simulink library "inp"  (R2021b)
settings: Solver=VariableStepAuto  StartTime=0.0  StopTime=10.0  RelTol=1e-3
undefined symbols (not defined in the file): C_TASK_5MS_S, FALSE, KINP_AcoreReadyToSlp_flg_ovrdflg, KINP_AcoreReadyToSlp_flg_ovrdval, KINP_AllowMovThd_OTA_enum_ovrdflg, KINP_AllowMovThd_OTA_enum_ovrdval, KINP_APSAngleTarget_Deg_ovrdflg, KINP_APSAngleTarget_Deg_ovrdval, KINP_APSDecReq_mps2_ovrdflg, KINP_APSDecReq_mps2_ovrdval, KINP_APSDecReqA_flg_ovrdflg, KINP_APSDecReqA_flg_ovrdval, KINP_APSDFLL_cm_ovrdflg, KINP_APSDFLL_cm_ovrdval, KINP_APSDFLR_cm_ovrdflg, KINP_APSDFLR_cm_ovrdval, KINP_APSDRLL_cm_ovrdflg, KINP_APSDRLL_cm_ovrdval, KINP_APSDRLR_cm_ovrdflg, KINP_APSDRLR_cm_ovrdval, KINP_APSExitCondition_enum_ovrdflg, KINP_APSExitCondition_enum_ovrdval, KINP_APSHWVer_enum_ovrdflg, KINP_APSHWVer_enum_ovrdval, KINP_APSProgressPCT_pct_ovrdflg, KINP_APSProgressPCT_pct_ovrdval, KINP_APSReq_enum_ovrdflg, KINP_APSReq_enum_ovrdval, KINP_APSRQDisplay_enum_ovrdflg, KINP_APSRQDisplay_enum_ovrdval, KINP_APSRqEPASCtrl_flg_ovrdflg, KINP_APSRqEPASCtrl_flg_ovrdval, KINP_APSShiftPosnReq_enum_ovrdval, KINP_APSShiftPosnReq_enum_ovrflg, KINP_APSSpeedCMD_kph_ovrdval, KINP_APSSpeedCMD_kph_ovrflg, KINP_APSStaSystem_enum_ovrdflg, KINP_APSStaSystem_enum_ovrdval, KINP_APSSWVer_enum_ovrdflg, KINP_APSSWVer_enum_ovrdval, KINP_APSVMCReqA_flg_ovrdval, KINP_APSVMCReqA_flg_ovrflg, KINP_APSVRqEPASCtrl_flg_ovrdflg, KINP_APSVRqEPASCtrl_flg_ovrdval, KINP_AuxBattVolmV_mV_ovrdflg, KINP_AuxBattVolmV_mV_ovrdval, KINP_CAASSta_enum_ovrdflg, KINP_CAASSta_enum_ovrdval, KINP_CAASVMCReqA_flg_ovrdval, KINP_CAASVMCReqA_flg_ovrflg, KINP_Chime_enum_ovrdflg, KINP_Chime_enum_ovrdval, KINP_ClearDTCcmd_flg_ovrdflg, KINP_ClearDTCcmd_flg_ovrdval, KINP_EvccAplusPwrUpReq_flg_ovrdflg, KINP_EvccAplusPwrUpReq_flg_ovrdval, KINP_LFID_raw_ovrdval, KINP_LFID_raw_ovrflg, KINP_LRID_raw_ovrdval, KINP_MemOffsetAccX_raw16_ovrdflg ... (+118)
libraries: FVT_lib x595, hcu_lib x1
(part 3 of 27)

== system inp/INP/APM/Subsystem7 ==
  In1 : Inport
  Constant : Constant  Value=KINP_PASDFCL_cm_ovrdval
  Constant1 : Constant  Value=KINP_PASDFCL_cm_ovrdflg
  Switch : Switch  Criteria=u2 ~= 0
  Out1 : Outport
  wires:
  Constant1/1 -> Switch/2
  Constant/1 -> Switch/1
  In1/1 -> Switch/3
  Switch/1 -> Out1/1

== system inp/INP/APM/Subsystem8 ==
  In1 : Inport
  Constant : Constant  Value=KINP_APSDRLR_cm_ovrdval
  Constant1 : Constant  Value=KINP_APSDRLR_cm_ovrdflg
  Switch : Switch  Criteria=u2 ~= 0
  Out1 : Outport
  wires:
  Switch/1 -> Out1/1
  In1/1 -> Switch/3
  Constant/1 -> Switch/1
  Constant1/1 -> Switch/2

== system inp/INP/APM/Subsystem9 ==
  In1 : Inport
  Constant : Constant  Value=KINP_APSDRLL_cm_ovrdval
  Constant1 : Constant  Value=KINP_APSDRLL_cm_ovrdflg
  Switch : Switch  Criteria=u2 ~= 0
  Out1 : Outport
  wires:
  Constant1/1 -> Switch/2
  Constant/1 -> Switch/1
  In1/1 -> Switch/3
  Switch/1 -> Out1/1

== system inp/INP/CAN1/CommunicationCheck ==
  BHAL_outputs : Inport
  CANMsgInvalidABM1 : FVT_lib/inp/CAN_Msg_Validity_Process_template  SystemSampleTime=-1  VariantActivationTime=update diagram  Latency=0  AutoFrameSizeCalculation=off
      link override debdec: Value=KINP_CANMsgInvalidABM1_flg_debdec
      link override debinc: Value=KINP_CANMsgInvalidABM1_flg_debinc
      link override deblim: Value=KINP_CANMsgInvalidABM1_flg_deblim
      link override inverse: Value=KINP_CANMsgInvalidABM1_flg_inverse
      link override ovrdflg: Value=KINP_CANMsgInvalidABM1_flg_ovrdflg
      link override ovrdval: Value=KINP_CANMsgInvalidABM1_flg_ovrdval
      link override srvcflg: Value=KINP_CANMsgInvalidABM1_flg_srvcflg
      link override srvcval: Value=KINP_CANMsgInvalidABM1_flg_srvcval
  CANMsgInvalidEPAS1 : FVT_lib/inp/CAN_Msg_Validity_Process_template  SystemSampleTime=-1  VariantActivationTime=update diagram  Latency=0  AutoFrameSizeCalculation=off
      link override debdec: Value=KINP_CANMsgInvalidEPAS1_flg_debdec
      link override debinc: Value=KINP_CANMsgInvalidEPAS1_flg_debinc
      link override deblim: Value=KINP_CANMsgInvalidEPAS1_flg_deblim
      link override inverse: Value=KINP_CANMsgInvalidEPAS1_flg_inverse
      link override ovrdflg: Value=KINP_CANMsgInvalidEPAS1_flg_ovrdflg
      link override ovrdval: Value=KINP_CANMsgInvalidEPAS1_flg_ovrdval
      link override srvcflg: Value=KINP_CANMsgInvalidEPAS1_flg_srvcflg
      link override srvcval: Value=KINP_CANMsgInvalidEPAS1_flg_srvcval
  CANMsgInvalidEPAS2 : FVT_lib/inp/CAN_Msg_Validity_Process_template  SystemSampleTime=-1  VariantActivationTime=update diagram  Latency=0  AutoFrameSizeCalculation=off
      link override debdec: Value=KINP_CANMsgInvalidEPAS2_flg_debdec
      link override debinc: Value=KINP_CANMsgInvalidEPAS2_flg_debinc
      link override deblim: Value=KINP_CANMsgInvalidEPAS2_flg_deblim
      link override inverse: Value=KINP_CANMsgInvalidEPAS2_flg_inverse
      link override ovrdflg: Value=KINP_CANMsgInvalidEPAS2_flg_ovrdflg
      link override ovrdval: Value=KINP_CANMsgInvalidEPAS2_flg_ovrdval
      link override srvcflg: Value=KINP_CANMsgInvalidEPAS2_flg_srvcflg
      link override srvcval: Value=KINP_CANMsgInvalidEPAS2_flg_srvcval
  CANMsgInvalidEPB1 : FVT_lib/inp/CAN_Msg_Validity_Process_template  SystemSampleTime=-1  VariantActivationTime=update diagram  Latency=0  AutoFrameSizeCalculation=off
      link override debdec: Value=KINP_CANMsgInvalidEPB1_flg_debdec
      link override debinc: Value=KINP_CANMsgInvalidEPB1_flg_debinc
      link override deblim: Value=KINP_CANMsgInvalidEPB1_flg_deblim
      link override inverse: Value=KINP_CANMsgInvalidEPB1_flg_inverse
      link override ovrdflg: Value=KINP_CANMsgInvalidEPB1_flg_ovrdflg
      link override ovrdval: Value=KINP_CANMsgInvalidEPB1_flg_ovrdval
      link override srvcflg: Value=KINP_CANMsgInvalidEPB1_flg_srvcflg
      link override srvcval: Value=KINP_CANMsgInvalidEPB1_flg_srvcval
  CANMsgInvalidESC1 : FVT_lib/inp/CAN_Msg_Validity_Process_template  SystemSampleTime=-1  VariantActivationTime=update diagram  Latency=0  AutoFrameSizeCalculation=off
      link override debdec: Value=KINP_CANMsgInvalidESC1_flg_debdec
      link override debinc: Value=KINP_CANMsgInvalidESC1_flg_debinc
      link override deblim: Value=KINP_CANMsgInvalidESC1_flg_deblim
      link override inverse: Value=KINP_CANMsgInvalidESC1_flg_inverse
      link override ovrdflg: Value=KINP_CANMsgInvalidESC1_flg_ovrdflg
      link override ovrdval: Value=KINP_CANMsgInvalidESC1_flg_ovrdval
      link override srvcflg: Value=KINP_CANMsgInvalidESC1_flg_srvcflg
      link override srvcval: Value=KINP_CANMsgInvalidESC1_flg_srvcval
  CANMsgInvalidESC2 : FVT_lib/inp/CAN_Msg_Validity_Process_template  SystemSampleTime=-1  VariantActivationTime=update diagram  Latency=0  AutoFrameSizeCalculation=off
      link override debdec: Value=KINP_CANMsgInvalidESC2_flg_debdec
      link override debinc: Value=KINP_CANMsgInvalidESC2_flg_debinc
      link override deblim: Value=KINP_CANMsgInvalidESC2_flg_deblim
      link override inverse: Value=KINP_CANMsgInvalidESC2_flg_inverse
      link override ovrdflg: Value=KINP_CANMsgInvalidESC2_flg_ovrdflg
      link override ovrdval: Value=KINP_CANMsgInvalidESC2_flg_ovrdval
      link override srvcflg: Value=KINP_CANMsgInvalidESC2_flg_srvcflg
      link override srvcval: Value=KINP_CANMsgInvalidESC2_flg_srvcval
  CANMsgInvalidESC3 : FVT_lib/inp/CAN_Msg_Validity_Process_template  SystemSampleTime=-1  VariantActivationTime=update diagram  Latency=0  AutoFrameSizeCalculation=off
      link override debdec: Value=KINP_CANMsgInvalidESC3_flg_debdec
      link override debinc: Value=KINP_CANMsgInvalidESC3_flg_debinc
      link override deblim: Value=KINP_CANMsgInvalidESC3_flg_deblim
      link override inverse: Value=KINP_CANMsgInvalidESC3_flg_inverse
      link override ovrdflg: Value=KINP_CANMsgInvalidESC3_flg_ovrdflg
      link override ovrdval: Value=KINP_CANMsgInvalidESC3_flg_ovrdval
      link override srvcflg: Value=KINP_CANMsgInvalidESC3_flg_srvcflg
      link override srvcval: Value=KINP_CANMsgInvalidESC3_flg_srvcval
  CANMsgInvalidESC4 : FVT_lib/inp/CAN_Msg_Validity_Process_template  SystemSampleTime=-1  VariantActivationTime=update diagram  Latency=0  AutoFrameSizeCalculation=off
      link override debdec: Value=KINP_CANMsgInvalidESC4_flg_debdec
      link override debinc: Value=KINP_CANMsgInvalidESC4_flg_debinc
      link override deblim: Value=KINP_CANMsgInvalidESC4_flg_deblim
      link override inverse: Value=KINP_CANMsgInvalidESC4_flg_inverse
      link override ovrdflg: Value=KINP_CANMsgInvalidESC4_flg_ovrdflg
      link override ovrdval: Value=KINP_CANMsgInvalidESC4_flg_ovrdval
      link override srvcflg: Value=KINP_CANMsgInvalidESC4_flg_srvcflg
      link override srvcval: Value=KINP_CANMsgInvalidESC4_flg_srvcval
  CANMsgInvalidESC5 : FVT_lib/inp/CAN_Msg_Validity_Process_template  SystemSampleTime=-1  VariantActivationTime=update diagram  Latency=0  AutoFrameSizeCalculation=off
      link override debdec: Value=KINP_CANMsgInvalidESC5_flg_debdec
      link override debinc: Value=KINP_CANMsgInvalidESC5_flg_debinc
      link override deblim: Value=KINP_CANMsgInvalidESC5_flg_deblim
      link override inverse: Value=KINP_CANMsgInvalidESC5_flg_inverse
      link override ovrdflg: Value=KINP_CANMsgInvalidESC5_flg_ovrdflg
      link override ovrdval: Value=KINP_CANMsgInvalidESC5_flg_ovrdval
      link override srvcflg: Value=KINP_CANMsgInvalidESC5_flg_srvcflg
      link override srvcval: Value=KINP_CANMsgInvalidESC5_flg_srvcval
  CANMsgInvalidESC6 : FVT_lib/inp/CAN_Msg_Validity_Process_template  SystemSampleTime=-1  VariantActivationTime=update diagram  Latency=0  AutoFrameSizeCalculation=off
      link override debdec: Value=KINP_CANMsgInvalidESC6_flg_debdec
      link override debinc: Value=KINP_CANMsgInvalidESC6_flg_debinc
      link override deblim: Value=KINP_CANMsgInvalidESC6_flg_deblim
      link override inverse: Value=KINP_CANMsgInvalidESC6_flg_inverse
      link override ovrdflg: Value=KINP_CANMsgInvalidESC6_flg_ovrdflg
      link override ovrdval: Value=KINP_CANMsgInvalidESC6_flg_ovrdval
      link override srvcflg: Value=KINP_CANMsgInvalidESC6_flg_srvcflg
      link override srvcval: Value=KINP_CANMsgInvalidESC6_flg_srvcval
  CANMsgInvalidESC7 : FVT_lib/inp/CAN_Msg_Validity_Process_template  SystemSampleTime=-1  VariantActivationTime=update diagram  Latency=0  AutoFrameSizeCalculation=off
      link override debdec: Value=KINP_CANMsgInvalidESC7_flg_debdec
      link override debinc: Value=KINP_CANMsgInvalidESC7_flg_debinc
      link override deblim: Value=KINP_CANMsgInvalidESC7_flg_deblim
      link override inverse: Value=KINP_CANMsgInvalidESC7_flg_inverse
      link override ovrdflg: Value=KINP_CANMsgInvalidESC7_flg_ovrdflg
      link override ovrdval: Value=KINP_CANMsgInvalidESC7_flg_ovrdval
      link override srvcflg: Value=KINP_CANMsgInvalidESC7_flg_srvcflg
      link override srvcval: Value=KINP_CANMsgInvalidESC7_flg_srvcval
  CANMsgInvalidFCM2 : FVT_lib/inp/CAN_Msg_Validity_Process_template  SystemSampleTime=-1  VariantActivationTime=update diagram  Latency=0  AutoFrameSizeCalculation=off
      link override debdec: Value=KINP_CANMsgInvalidFCM2_flg_debdec
      link override debinc: Value=KINP_CANMsgInvalidFCM2_flg_debinc
      link override deblim: Value=KINP_CANMsgInvalidFCM2_flg_deblim
      link override inverse: Value=KINP_CANMsgInvalidFCM2_flg_inverse
      link override ovrdflg: Value=KINP_CANMsgInvalidFCM2_flg_ovrdflg
      link override ovrdval: Value=KINP_CANMsgInvalidFCM2_flg_ovrdval
      link override srvcflg: Value=KINP_CANMsgInvalidFCM2_flg_srvcflg
      link override srvcval: Value=KINP_CANMsgInvalidFCM2_flg_srvcval
  CANMsgInvalidFCM3 : FVT_lib/inp/CAN_Msg_Validity_Process_template  SystemSampleTime=-1  VariantActivationTime=update diagram  Latency=0  AutoFrameSizeCalculation=off
      link override debdec: Value=KINP_CANMsgInvalidFCM3_flg_debdec
      link override debinc: Value=KINP_CANMsgInvalidFCM3_flg_debinc
      link override deblim: Value=KINP_CANMsgInvalidFCM3_flg_deblim
      link override inverse: Value=KINP_CANMsgInvalidFCM3_flg_inverse
      link override ovrdflg: Value=KINP_CANMsgInvalidFCM3_flg_ovrdflg
      link override ovrdval: Value=KINP_CANMsgInvalidFCM3_flg_ovrdval
      link override srvcflg: Value=KINP_CANMsgInvalidFCM3_flg_srvcflg
      link override srvcval: Value=KINP_CANMsgInvalidFCM3_flg_srvcval
  CANMsgInvalidFCM4 : FVT_lib/inp/CAN_Msg_Validity_Process_template  SystemSampleTime=-1  VariantActivationTime=update diagram  Latency=0  AutoFrameSizeCalculation=off
      link override debdec: Value=KINP_CANMsgInvalidFCM4_flg_debdec
      link override debinc: Value=KINP_CANMsgInvalidFCM4_flg_debinc
      link override deblim: Value=KINP_CANMsgInvalidFCM4_flg_deblim
      link override inverse: Value=KINP_CANMsgInvalidFCM4_flg_inverse
      link override ovrdflg: Value=KINP_CANMsgInvalidFCM4_flg_ovrdflg
      link override ovrdval: Value=KINP_CANMsgInvalidFCM4_flg_ovrdval
      link override srvcflg: Value=KINP_CANMsgInvalidFCM4_flg_srvcflg
      link override srvcval: Value=KINP_CANMsgInvalidFCM4_flg_srvcval
  CANMsgInvalidSRR1 : FVT_lib/inp/CAN_Msg_Validity_Process_template  SystemSampleTime=-1  VariantActivationTime=update diagram  Latency=0  AutoFrameSizeCalculation=off
      link override debdec: Value=KINP_CANMsgInvalidSRR1_flg_debdec
      link override debinc: Value=KINP_CANMsgInvalidSRR1_flg_debinc
      link override deblim: Value=KINP_CANMsgInvalidSRR1_flg_deblim
      link override inverse: Value=KINP_CANMsgInvalidSRR1_flg_inverse
      link override ovrdflg: Value=KINP_CANMsgInvalidSRR1_flg_ovrdflg
      link override ovrdval: Value=KINP_CANMsgInvalidSRR1_flg_ovrdval
      link override srvcflg: Value=KINP_CANMsgInvalidSRR1_flg_srvcflg
      link override srvcval: Value=KINP_CANMsgInvalidSRR1_flg_srvcval
  bus_creator : BusCreator  Inputs=15
  bus_selector : BusSelector  OutputSignals=VHAL_CANMsgInvalidABM1_flg,VHAL_CANMsgInvalidEPAS1_flg,VHAL_CANMsgInvalidEPAS2_flg,VHAL_CANMsgInvalidEPB1_flg,VHAL_CANMsgInvalidESC1_flg,VHAL_CANMsgInvalidESC2_flg,VHAL_CANMsgInvalidESC3_flg,VHAL_CANMsgInvalidESC4_flg,VHAL_CANMsgInvalidESC5_flg,VHAL_CANMsgInvalidESC6_flg,VHAL_CANMsgInvalidESC7_flg,VHAL_CANMsgInvalidFCM2_flg,VHAL_CANMsgInvalidFCM3_flg,VHAL_CANMsgInvalidFCM4_flg,VHAL_CANMsgInvalidSRR1_flg
  not{1..15} (15 alike) : Logic  Operator=NOT  AllPortsSameDT=off  OutDataTypeStr=boolean
  inp_CanValid_bus : Outport
  wires:
  BHAL_outputs/1 -> [BHAL_outputs]
  bus_selector/1 -> CANMsgInvalidABM1/1  "<VHAL_CANMsgInvalidABM1_flg>"
  CANMsgInvalidABM1/1 -> not1/1
  not1/1 -> bus_creator/1  "VINP_CANMsgValidABM1_flg"
  bus_selector/2 -> CANMsgInvalidEPAS1/1  "<VHAL_CANMsgInvalidEPAS1_flg>"
  CANMsgInvalidEPAS1/1 -> not2/1
  not2/1 -> bus_creator/2  "VINP_CANMsgValidEPAS1_flg"
  bus_selector/3 -> CANMsgInvalidEPAS2/1  "<VHAL_CANMsgInvalidEPAS2_flg>"
  CANMsgInvalidEPAS2/1 -> not3/1
  not3/1 -> bus_creator/3  "VINP_CANMsgValidEPAS2_flg"
  bus_selector/4 -> CANMsgInvalidEPB1/1  "<VHAL_CANMsgInvalidEPB1_flg>"
  CANMsgInvalidEPB1/1 -> not4/1
  not4/1 -> bus_creator/4  "VINP_CANMsgValidEPB1_flg"
  bus_selector/5 -> CANMsgInvalidESC1/1  "<VHAL_CANMsgInvalidESC1_flg>"
  CANMsgInvalidESC1/1 -> not5/1
  not5/1 -> bus_creator/5  "VINP_CANMsgValidESC1_flg"
  bus_selector/6 -> CANMsgInvalidESC2/1  "<VHAL_CANMsgInvalidESC2_flg>"
  CANMsgInvalidESC2/1 -> not6/1
  not6/1 -> bus_creator/6  "VINP_CANMsgValidESC2_flg"
  bus_selector/7 -> CANMsgInvalidESC3/1  "<VHAL_CANMsgInvalidESC3_flg>"
  CANMsgInvalidESC3/1 -> not7/1
  not7/1 -> bus_creator/7  "VINP_CANMsgValidESC3_flg"
  bus_selector/8 -> CANMsgInvalidESC4/1  "<VHAL_CANMsgInvalidESC4_flg>"
  CANMsgInvalidESC4/1 -> not8/1
  not8/1 -> bus_creator/8  "VINP_CANMsgValidESC4_flg"
  bus_selector/9 -> CANMsgInvalidESC5/1  "<VHAL_CANMsgInvalidESC5_flg>"
  CANMsgInvalidESC5/1 -> not9/1
  not9/1 -> bus_creator/9  "VINP_CANMsgValidESC5_flg"
  bus_selector/10 -> CANMsgInvalidESC6/1  "<VHAL_CANMsgInvalidESC6_flg>"
  CANMsgInvalidESC6/1 -> not10/1
  not10/1 -> bus_creator/10  "VINP_CANMsgValidESC6_flg"
  bus_selector/11 -> CANMsgInvalidESC7/1  "<VHAL_CANMsgInvalidESC7_flg>"
  CANMsgInvalidESC7/1 -> not11/1
  not11/1 -> bus_creator/11  "VINP_CANMsgValidESC7_flg"
  bus_selector/12 -> CANMsgInvalidFCM2/1  "<VHAL_CANMsgInvalidFCM2_flg>"
  CANMsgInvalidFCM2/1 -> not12/1
  not12/1 -> bus_creator/12  "VINP_CANMsgValidFCM2_flg"
  bus_selector/13 -> CANMsgInvalidFCM3/1  "<VHAL_CANMsgInvalidFCM3_flg>"
  CANMsgInvalidFCM3/1 -> not13/1
  not13/1 -> bus_creator/13  "VINP_CANMsgValidFCM3_flg"
  bus_selector/14 -> CANMsgInvalidFCM4/1  "<VHAL_CANMsgInvalidFCM4_flg>"
  CANMsgInvalidFCM4/1 -> not14/1
  not14/1 -> bus_creator/14  "VINP_CANMsgValidFCM4_flg"
  bus_selector/15 -> CANMsgInvalidSRR1/1  "<VHAL_CANMsgInvalidSRR1_flg>"
  CANMsgInvalidSRR1/1 -> not15/1
  not15/1 -> bus_creator/15  "VINP_CANMsgValidSRR1_flg"
  [BHAL_outputs] -> bus_selector/1
  bus_creator/1 -> inp_CanValid_bus/1

== system inp/INP/CAN1/CreateBus ==
  inp_CanValid_bus : Inport
  inp_Hal_bus : Inport  Port=2
  UnitConverter_{1..18,21,23..26,30,32..35,37..38,40..41,44,47,50,52,55,57,60,62,65,67,69..78,80..92,96,98,100,102..103,106..108,110,113,117..119,121,124..125,128,131..132,138..140} (87 alike) : DataTypeConversion  OutDataTypeStr=boolean
  UnitConverter_{29,31,45..46,48,51,56,61,66,79,95,97,99,101,109,114,116,120,126..127} (20 alike) : DataTypeConversion  OutDataTypeStr=single
  UnitConverter_{19..20,22,27..28,36,39,42..43,49,53..54,58..59,63..64,68,93..94,104..105,111..112,115,122..123,129..130,133..137,141..146} (39 alike) : DataTypeConversion  OutDataTypeStr=uint8
  bus_creator : BusCreator  Inputs=146
  bus_selector : BusSelector  OutputSignals=VINP_CANMsgValidABM1_flg,VINP_CANMsgValidEPAS1_flg,VINP_CANMsgValidEPAS2_flg,VINP_CANMsgValidEPB1_flg,VINP_CANMsgValidESC1_flg,VINP_CANMsgValidESC2_flg,VINP_CANMsgValidESC3_flg,VINP_CANMsgValidESC4_flg,VINP_CANMsgValidESC5_flg,VINP_CANMsgValidESC6_flg,VINP_CANMsgValidESC7_flg,VINP_CANMsgValidFCM2_flg,VINP_CANMsgValidFCM3_flg,VINP_CANMsgValidFCM4_flg,VINP_CANMsgValidSRR1_flg
  bus_selector_1 : BusSelector  OutputSignals=VINP_ABM1CSErr_flg,VINP_ABM1RCErr_flg,VINP_AirBagFailCmd_flg,VINP_ChecksumABM1_enum,VINP_CrashOutputSts_enum,VINP_DriverSeatBeltCmd_flg,VINP_LifeCountABM1_enum,VINP_PsngrSeatBeltCmd_flg,VINP_RCenterSeatBeltCmd_flg,VINP_RDriverSeatBeltCmd_flg,VINP_RPsngrSeatBeltCmd_flg,VINP_DriIntend_enum,VINP_EPSAOIControl_enum,VINP_SASAngle_Deg,VINP_SASCAL_flg,VINP_SASSpeed_degps,VINP_SASSpeedValid_flg,VINP_SASV_flg,VINP_DOASta_flg,VINP_EPBCarWashMode_flg,VINP_EPBErrSta_enum,VINP_EPBExtApplyAvail_flg,VINP_EPBExtReleaseAvail_flg,VINP_EPBSta_enum,VINP_ESC1CSErr_flg,VINP_ESC1RCErr_flg,VINP_ESC1CS_enum,VINP_ESC1RC_enum,VINP_FrPTCSActive_flg,VINP_FrntAxlTrqReqDrv_Nm,VINP_RearAxlTrqReqDrv_Nm,VINP_RrPTCSActive_flg,VINP_VehSpeed_kph,VINP_LFPulseCount_enum,VINP_LFPulseCountV_flg,VINP_LFRawWhlSpeed_kph,VINP_LFRawWhlSpeedV_flg,VINP_LFWhlRotDir_enum,VINP_RFPulseCount_enum,VINP_RFPulseCountV_flg,VINP_RFRawWhlSpeed_kph,VINP_RFRawWhlSpeedV_flg,VINP_RFWhlRotDir_enum,VINP_LRPulseCount_enum,VINP_LRPulseCountV_flg,VINP_LRRawWhlSpeed_kph,VINP_LRRawWhlSpeedV_flg,VINP_LRWhlRotDir_enum,VINP_RRPulseCount_enum,VINP_RRPulseCountV_flg,VINP_RRRawWhlSpeed_kph,VINP_RRRawWhlSpeedV_flg,VINP_RRWhlRotDir_enum,VINP_ABSActive_flg,VINP_ABSFailed_flg,VINP_AVHActive_flg,VINP_AVHFailed_flg,VINP_BTCSActive_flg,VINP_EBDActive_flg,VINP_EBDFailed_flg,VINP_ESCActive_flg,VINP_ESCFailed_flg,VINP_ESSActive_flg,VINP_GRADE_Deg,VINP_HBBActive_flg,VINP_HBBFailed_flg,VINP_HDDActive_flg,VINP_HDDFailed_flg,VINP_HSAActive_flg,VINP_HSAFailed_flg,VINP_PBAFailed_flg,VINP_TCSActive_flg,VINP_TCSFailed_flg,VINP_ESC5CSErr_flg,VINP_ESC5RCErr_flg,VINP_BrkSwSta_flg,VINP_BrkSwV_flg,VINP_ESC5CRC8_enum,VINP_ESC5RC_enum,VINP_LatAccel_Gps,VINP_LatAccelV_flg,VINP_LongAccel_Gps,VINP_LongAccelV_flg,VINP_MCPressure_bar,VINP_MCPressureV_flg,VINP_YawRate_degps,VINP_YawRateV_flg,VINP_ActBrkLampSta_flg,VINP_ESCADASSta_enum,VINP_ESCAPSSta_enum,VINP_ESCStandstill_flg,VINP_ESC7CSErr_flg,VINP_ESC7RCErr_flg,VINP_BrkPedalPos_pct,VINP_BrkPedalPosSta_flg,VINP_ESC7CS_enum,VINP_ESC7RC_enum,VINP_FrRBCActive_flg,VINP_FrntAxlTrqReqBrk_Nm,VINP_RDCActive_enum,VINP_RearAxlTrqReqBrk_Nm,VINP_RrRBCActive_flg,VINP_FCM2CSErr_flg,VINP_FCM2RCErr_flg,VINP_ACCRequiredAccel_mps2,VINP_ACCVehHoldReq_flg,VINP_FCM2Checksum_enum,VINP_FCM2LifeCount_enum,VINP_FCM3CSErr_flg,VINP_FCM3RCErr_flg,VINP_ACCObjDist_m,VINP_ACCObjRelSpd_mps,VINP_ADASForceIdle_flg,VINP_FCM3Checksum_enum,VINP_FCM3LifeCount_enum,VINP_FCM4CSErr_flg,VINP_FCM4RCErr_flg,VINP_ACCSetSpeed_enum,VINP_ACCSetSpeedDisp_enum,VINP_ADASACCSta_enum,VINP_FCM4Checksum_enum,VINP_ForceLowBeam_enum,VINP_HazardWarningReq_flg,VINP_LeftTurnLightReq_flg,VINP_RightTurnLightReq_flg,VINP_TargetType_enum,VINP_TimeGapLevel_enum,VINP_SRRBSDWarnL_enum,VINP_SRRBSDWarnR_enum,VINP_SRRODAWarnL_enum,VINP_SRRODAWarnR_enum
  BINP_outputs : Outport
  wires:
  inp_CanValid_bus/1 -> [inp_CanValid_bus]
  inp_Hal_bus/1 -> [inp_Hal_bus]
  bus_selector/1 -> UnitConverter_1/1  "<VINP_CANMsgValidABM1_flg>"
  UnitConverter_1/1 -> bus_creator/1  "VINP_CANMsgValidABM1_flg"
  bus_selector/2 -> UnitConverter_2/1  "<VINP_CANMsgValidEPAS1_flg>"
  UnitConverter_2/1 -> bus_creator/2  "VINP_CANMsgValidEPAS1_flg"
  bus_selector/3 -> UnitConverter_3/1  "<VINP_CANMsgValidEPAS2_flg>"
  UnitConverter_3/1 -> bus_creator/3  "VINP_CANMsgValidEPAS2_flg"
  bus_selector/4 -> UnitConverter_4/1  "<VINP_CANMsgValidEPB1_flg>"
  UnitConverter_4/1 -> bus_creator/4  "VINP_CANMsgValidEPB1_flg"
  bus_selector/5 -> UnitConverter_5/1  "<VINP_CANMsgValidESC1_flg>"
  UnitConverter_5/1 -> bus_creator/5  "VINP_CANMsgValidESC1_flg"
  bus_selector/6 -> UnitConverter_6/1  "<VINP_CANMsgValidESC2_flg>"
  UnitConverter_6/1 -> bus_creator/6  "VINP_CANMsgValidESC2_flg"
  bus_selector/7 -> UnitConverter_7/1  "<VINP_CANMsgValidESC3_flg>"
  UnitConverter_7/1 -> bus_creator/7  "VINP_CANMsgValidESC3_flg"
  bus_selector/8 -> UnitConverter_8/1  "<VINP_CANMsgValidESC4_flg>"
  UnitConverter_8/1 -> bus_creator/8  "VINP_CANMsgValidESC4_flg"
  bus_selector/9 -> UnitConverter_9/1  "<VINP_CANMsgValidESC5_flg>"
  UnitConverter_9/1 -> bus_creator/9  "VINP_CANMsgValidESC5_flg"
  bus_selector/10 -> UnitConverter_10/1  "<VINP_CANMsgValidESC6_flg>"
  UnitConverter_10/1 -> bus_creator/10  "VINP_CANMsgValidESC6_flg"
  bus_selector/11 -> UnitConverter_11/1  "<VINP_CANMsgValidESC7_flg>"
  UnitConverter_11/1 -> bus_creator/11  "VINP_CANMsgValidESC7_flg"
  bus_selector/12 -> UnitConverter_12/1  "<VINP_CANMsgValidFCM2_flg>"
  UnitConverter_12/1 -> bus_creator/12  "VINP_CANMsgValidFCM2_flg"
  bus_selector/13 -> UnitConverter_13/1  "<VINP_CANMsgValidFCM3_flg>"
  UnitConverter_13/1 -> bus_creator/13  "VINP_CANMsgValidFCM3_flg"
  bus_selector/14 -> UnitConverter_14/1  "<VINP_CANMsgValidFCM4_flg>"
  UnitConverter_14/1 -> bus_creator/14  "VINP_CANMsgValidFCM4_flg"
  bus_selector/15 -> UnitConverter_15/1  "<VINP_CANMsgValidSRR1_flg>"
  UnitConverter_15/1 -> bus_creator/15  "VINP_CANMsgValidSRR1_flg"
  bus_selector_1/1 -> UnitConverter_16/1  "<VINP_ABM1CSErr_flg>"
  UnitConverter_16/1 -> bus_creator/16  "VINP_ABM1CSErr_flg"
  bus_selector_1/2 -> UnitConverter_17/1  "<VINP_ABM1RCErr_flg>"
  UnitConverter_17/1 -> bus_creator/17  "VINP_ABM1RCErr_flg"
  bus_selector_1/3 -> UnitConverter_18/1  "<VINP_AirBagFailCmd_flg>"
  UnitConverter_18/1 -> bus_creator/18  "VINP_AirBagFailCmd_flg"
  bus_selector_1/4 -> UnitConverter_19/1  "<VINP_ChecksumABM1_enum>"
  UnitConverter_19/1 -> bus_creator/19  "VINP_ChecksumABM1_enum"
  bus_selector_1/5 -> UnitConverter_20/1  "<VINP_CrashOutputSts_enum>"
  UnitConverter_20/1 -> bus_creator/20  "VINP_CrashOutputSts_enum"
  bus_selector_1/6 -> UnitConverter_21/1  "<VINP_DriverSeatBeltCmd_flg>"
  UnitConverter_21/1 -> bus_creator/21  "VINP_DriverSeatBeltCmd_flg"
  bus_selector_1/7 -> UnitConverter_22/1  "<VINP_LifeCountABM1_enum>"
  UnitConverter_22/1 -> bus_creator/22  "VINP_LifeCountABM1_enum"
  bus_selector_1/8 -> UnitConverter_23/1  "<VINP_PsngrSeatBeltCmd_flg>"
  UnitConverter_23/1 -> bus_creator/23  "VINP_PsngrSeatBeltCmd_flg"
  bus_selector_1/9 -> UnitConverter_24/1  "<VINP_RCenterSeatBeltCmd_flg>"
  UnitConverter_24/1 -> bus_creator/24  "VINP_RCenterSeatBeltCmd_flg"
  bus_selector_1/10 -> UnitConverter_25/1  "<VINP_RDriverSeatBeltCmd_flg>"
  UnitConverter_25/1 -> bus_creator/25  "VINP_RDriverSeatBeltCmd_flg"
  bus_selector_1/11 -> UnitConverter_26/1  "<VINP_RPsngrSeatBeltCmd_flg>"
  UnitConverter_26/1 -> bus_creator/26  "VINP_RPsngrSeatBeltCmd_flg"
  bus_selector_1/12 -> UnitConverter_27/1  "<VINP_DriIntend_enum>"
  UnitConverter_27/1 -> bus_creator/27  "VINP_DriIntend_enum"
  bus_selector_1/13 -> UnitConverter_28/1  "<VINP_EPSAOIControl_enum>"
  UnitConverter_28/1 -> bus_creator/28  "VINP_EPSAOIControl_enum"
  bus_selector_1/14 -> UnitConverter_29/1  "<VINP_SASAngle_Deg>"
  UnitConverter_29/1 -> bus_creator/29  "VINP_SASAngle_Deg"
  bus_selector_1/15 -> UnitConverter_30/1  "<VINP_SASCAL_flg>"
  UnitConverter_30/1 -> bus_creator/30  "VINP_SASCAL_flg"
  bus_selector_1/16 -> UnitConverter_31/1  "<VINP_SASSpeed_degps>"
  UnitConverter_31/1 -> bus_creator/31  "VINP_SASSpeed_degps"
  bus_selector_1/17 -> UnitConverter_32/1  "<VINP_SASSpeedValid_flg>"
  UnitConverter_32/1 -> bus_creator/32  "VINP_SASSpeedValid_flg"
  bus_selector_1/18 -> UnitConverter_33/1  "<VINP_SASV_flg>"
  UnitConverter_33/1 -> bus_creator/33  "VINP_SASV_flg"
  bus_selector_1/19 -> UnitConverter_34/1  "<VINP_DOASta_flg>"
  UnitConverter_34/1 -> bus_creator/34  "VINP_DOASta_flg"
  bus_selector_1/20 -> UnitConverter_35/1  "<VINP_EPBCarWashMode_flg>"
  UnitConverter_35/1 -> bus_creator/35  "VINP_EPBCarWashMode_flg"
  bus_selector_1/21 -> UnitConverter_36/1  "<VINP_EPBErrSta_enum>"
  UnitConverter_36/1 -> bus_creator/36  "VINP_EPBErrSta_enum"
  bus_selector_1/22 -> UnitConverter_37/1  "<VINP_EPBExtApplyAvail_flg>"
  UnitConverter_37/1 -> bus_creator/37  "VINP_EPBExtApplyAvail_flg"
  bus_selector_1/23 -> UnitConverter_38/1  "<VINP_EPBExtReleaseAvail_flg>"
  UnitConverter_38/1 -> bus_creator/38  "VINP_EPBExtReleaseAvail_flg"
  bus_selector_1/24 -> UnitConverter_39/1  "<VINP_EPBSta_enum>"
  UnitConverter_39/1 -> bus_creator/39  "VINP_EPBSta_enum"
  bus_selector_1/25 -> UnitConverter_40/1  "<VINP_ESC1CSErr_flg>"
  UnitConverter_40/1 -> bus_creator/40  "VINP_ESC1CSErr_flg"
  bus_selector_1/26 -> UnitConverter_41/1  "<VINP_ESC1RCErr_flg>"
  UnitConverter_41/1 -> bus_creator/41  "VINP_ESC1RCErr_flg"
  bus_selector_1/27 -> UnitConverter_42/1  "<VINP_ESC1CS_enum>"
  UnitConverter_42/1 -> bus_creator/42  "VINP_ESC1CS_enum"
  bus_selector_1/28 -> UnitConverter_43/1  "<VINP_ESC1RC_enum>"
  UnitConverter_43/1 -> bus_creator/43  "VINP_ESC1RC_enum"
  bus_selector_1/29 -> UnitConverter_44/1  "<VINP_FrPTCSActive_flg>"
  UnitConverter_44/1 -> bus_creator/44  "VINP_FrPTCSActive_flg"
  bus_selector_1/30 -> UnitConverter_45/1  "<VINP_FrntAxlTrqReqDrv_Nm>"
  UnitConverter_45/1 -> bus_creator/45  "VINP_FrntAxlTrqReqDrv_Nm"
  bus_selector_1/31 -> UnitConverter_46/1  "<VINP_RearAxlTrqReqDrv_Nm>"
  UnitConverter_46/1 -> bus_creator/46  "VINP_RearAxlTrqReqDrv_Nm"
  bus_selector_1/32 -> UnitConverter_47/1  "<VINP_RrPTCSActive_flg>"
  UnitConverter_47/1 -> bus_creator/47  "VINP_RrPTCSActive_flg"
  bus_selector_1/33 -> UnitConverter_48/1  "<VINP_VehSpeed_kph>"
  UnitConverter_48/1 -> bus_creator/48  "VINP_VehSpeed_kph"
  bus_selector_1/34 -> UnitConverter_49/1  "<VINP_LFPulseCount_enum>"
  UnitConverter_49/1 -> bus_creator/49  "VINP_LFPulseCount_enum"
  bus_selector_1/35 -> UnitConverter_50/1  "<VINP_LFPulseCountV_flg>"
  UnitConverter_50/1 -> bus_creator/50  "VINP_LFPulseCountV_flg"
  bus_selector_1/36 -> UnitConverter_51/1  "<VINP_LFRawWhlSpeed_kph>"
  UnitConverter_51/1 -> bus_creator/51  "VINP_LFRawWhlSpeed_kph"
  bus_selector_1/37 -> UnitConverter_52/1  "<VINP_LFRawWhlSpeedV_flg>"
  UnitConverter_52/1 -> bus_creator/52  "VINP_LFRawWhlSpeedV_flg"
  bus_selector_1/38 -> UnitConverter_53/1  "<VINP_LFWhlRotDir_enum>"
  UnitConverter_53/1 -> bus_creator/53  "VINP_LFWhlRotDir_enum"
  bus_selector_1/39 -> UnitConverter_54/1  "<VINP_RFPulseCount_enum>"
  UnitConverter_54/1 -> bus_creator/54  "VINP_RFPulseCount_enum"
  bus_selector_1/40 -> UnitConverter_55/1  "<VINP_RFPulseCountV_flg>"
  UnitConverter_55/1 -> bus_creator/55  "VINP_RFPulseCountV_flg"
  bus_selector_1/41 -> UnitConverter_56/1  "<VINP_RFRawWhlSpeed_kph>"
  UnitConverter_56/1 -> bus_creator/56  "VINP_RFRawWhlSpeed_kph"
  bus_selector_1/42 -> UnitConverter_57/1  "<VINP_RFRawWhlSpeedV_flg>"
  UnitConverter_57/1 -> bus_creator/57  "VINP_RFRawWhlSpeedV_flg"
  bus_selector_1/43 -> UnitConverter_58/1  "<VINP_RFWhlRotDir_enum>"
  UnitConverter_58/1 -> bus_creator/58  "VINP_RFWhlRotDir_enum"
  bus_selector_1/44 -> UnitConverter_59/1  "<VINP_LRPulseCount_enum>"
  UnitConverter_59/1 -> bus_creator/59  "VINP_LRPulseCount_enum"
  bus_selector_1/45 -> UnitConverter_60/1  "<VINP_LRPulseCountV_flg>"
  UnitConverter_60/1 -> bus_creator/60  "VINP_LRPulseCountV_flg"
  bus_selector_1/46 -> UnitConverter_61/1  "<VINP_LRRawWhlSpeed_kph>"
  UnitConverter_61/1 -> bus_creator/61  "VINP_LRRawWhlSpeed_kph"
  bus_selector_1/47 -> UnitConverter_62/1  "<VINP_LRRawWhlSpeedV_flg>"
  UnitConverter_62/1 -> bus_creator/62  "VINP_LRRawWhlSpeedV_flg"
  bus_selector_1/48 -> UnitConverter_63/1  "<VINP_LRWhlRotDir_enum>"
  UnitConverter_63/1 -> bus_creator/63  "VINP_LRWhlRotDir_enum"
  bus_selector_1/49 -> UnitConverter_64/1  "<VINP_RRPulseCount_enum>"
  UnitConverter_64/1 -> bus_creator/64  "VINP_RRPulseCount_enum"
  bus_selector_1/50 -> UnitConverter_65/1  "<VINP_RRPulseCountV_flg>"
  UnitConverter_65/1 -> bus_creator/65  "VINP_RRPulseCountV_flg"
  bus_selector_1/51 -> UnitConverter_66/1  "<VINP_RRRawWhlSpeed_kph>"
  UnitConverter_66/1 -> bus_creator/66  "VINP_RRRawWhlSpeed_kph"
  bus_selector_1/52 -> UnitConverter_67/1  "<VINP_RRRawWhlSpeedV_flg>"
  UnitConverter_67/1 -> bus_creator/67  "VINP_RRRawWhlSpeedV_flg"
  bus_selector_1/53 -> UnitConverter_68/1  "<VINP_RRWhlRotDir_enum>"
  UnitConverter_68/1 -> bus_creator/68  "VINP_RRWhlRotDir_enum"
  bus_selector_1/54 -> UnitConverter_69/1  "<VINP_ABSActive_flg>"
  UnitConverter_69/1 -> bus_creator/69  "VINP_ABSActive_flg"
  bus_selector_1/55 -> UnitConverter_70/1  "<VINP_ABSFailed_flg>"
  UnitConverter_70/1 -> bus_creator/70  "VINP_ABSFailed_flg"
  bus_selector_1/56 -> UnitConverter_71/1  "<VINP_AVHActive_flg>"
  UnitConverter_71/1 -> bus_creator/71  "VINP_AVHActive_flg"
  bus_selector_1/57 -> UnitConverter_72/1  "<VINP_AVHFailed_flg>"
  UnitConverter_72/1 -> bus_creator/72  "VINP_AVHFailed_flg"
  bus_selector_1/58 -> UnitConverter_73/1  "<VINP_BTCSActive_flg>"
  UnitConverter_73/1 -> bus_creator/73  "VINP_BTCSActive_flg"
  bus_selector_1/59 -> UnitConverter_74/1  "<VINP_EBDActive_flg>"
  UnitConverter_74/1 -> bus_creator/74  "VINP_EBDActive_flg"
  bus_selector_1/60 -> UnitConverter_75/1  "<VINP_EBDFailed_flg>"
  UnitConverter_75/1 -> bus_creator/75  "VINP_EBDFailed_flg"
  bus_selector_1/61 -> UnitConverter_76/1  "<VINP_ESCActive_flg>"
  UnitConverter_76/1 -> bus_creator/76  "VINP_ESCActive_flg"
  bus_selector_1/62 -> UnitConverter_77/1  "<VINP_ESCFailed_flg>"
  UnitConverter_77/1 -> bus_creator/77  "VINP_ESCFailed_flg"
  bus_selector_1/63 -> UnitConverter_78/1  "<VINP_ESSActive_flg>"
  UnitConverter_78/1 -> bus_creator/78  "VINP_ESSActive_flg"
  bus_selector_1/64 -> UnitConverter_79/1  "<VINP_GRADE_Deg>"
  UnitConverter_79/1 -> bus_creator/79  "VINP_GRADE_Deg"
  bus_selector_1/65 -> UnitConverter_80/1  "<VINP_HBBActive_flg>"
  UnitConverter_80/1 -> bus_creator/80  "VINP_HBBActive_flg"
  bus_selector_1/66 -> UnitConverter_81/1  "<VINP_HBBFailed_flg>"
  UnitConverter_81/1 -> bus_creator/81  "VINP_HBBFailed_flg"
  bus_selector_1/67 -> UnitConverter_82/1  "<VINP_HDDActive_flg>"
  UnitConverter_82/1 -> bus_creator/82  "VINP_HDDActive_flg"
  bus_selector_1/68 -> UnitConverter_83/1  "<VINP_HDDFailed_flg>"
  UnitConverter_83/1 -> bus_creator/83  "VINP_HDDFailed_flg"
  bus_selector_1/69 -> UnitConverter_84/1  "<VINP_HSAActive_flg>"
  UnitConverter_84/1 -> bus_creator/84  "VINP_HSAActive_flg"
  bus_selector_1/70 -> UnitConverter_85/1  "<VINP_HSAFailed_flg>"
  UnitConverter_85/1 -> bus_creator/85  "VINP_HSAFailed_flg"
  bus_selector_1/71 -> UnitConverter_86/1  "<VINP_PBAFailed_flg>"
  UnitConverter_86/1 -> bus_creator/86  "VINP_PBAFailed_flg"
  bus_selector_1/72 -> UnitConverter_87/1  "<VINP_TCSActive_flg>"
  UnitConverter_87/1 -> bus_creator/87  "VINP_TCSActive_flg"
  bus_selector_1/73 -> UnitConverter_88/1  "<VINP_TCSFailed_flg>"
  UnitConverter_88/1 -> bus_creator/88  "VINP_TCSFailed_flg"
  bus_selector_1/74 -> UnitConverter_89/1  "<VINP_ESC5CSErr_flg>"
  UnitConverter_89/1 -> bus_creator/89  "VINP_ESC5CSErr_flg"
  bus_selector_1/75 -> UnitConverter_90/1  "<VINP_ESC5RCErr_flg>"
  UnitConverter_90/1 -> bus_creator/90  "VINP_ESC5RCErr_flg"
  bus_selector_1/76 -> UnitConverter_91/1  "<VINP_BrkSwSta_flg>"
  UnitConverter_91/1 -> bus_creator/91  "VINP_BrkSwSta_flg"
  bus_selector_1/77 -> UnitConverter_92/1  "<VINP_BrkSwV_flg>"
  UnitConverter_92/1 -> bus_creator/92  "VINP_BrkSwV_flg"
  bus_selector_1/78 -> UnitConverter_93/1  "<VINP_ESC5CRC8_enum>"
  UnitConverter_93/1 -> bus_creator/93  "VINP_ESC5CRC8_enum"
  bus_selector_1/79 -> UnitConverter_94/1  "<VINP_ESC5RC_enum>"
  UnitConverter_94/1 -> bus_creator/94  "VINP_ESC5RC_enum"
  bus_selector_1/80 -> UnitConverter_95/1  "<VINP_LatAccel_Gps>"
  UnitConverter_95/1 -> bus_creator/95  "VINP_LatAccel_Gps"
  bus_selector_1/81 -> UnitConverter_96/1  "<VINP_LatAccelV_flg>"
  UnitConverter_96/1 -> bus_creator/96  "VINP_LatAccelV_flg"
  bus_selector_1/82 -> UnitConverter_97/1  "<VINP_LongAccel_Gps>"
  UnitConverter_97/1 -> bus_creator/97  "VINP_LongAccel_Gps"
  bus_selector_1/83 -> UnitConverter_98/1  "<VINP_LongAccelV_flg>"
  UnitConverter_98/1 -> bus_creator/98  "VINP_LongAccelV_flg"
  bus_selector_1/84 -> UnitConverter_99/1  "<VINP_MCPressure_bar>"
  UnitConverter_99/1 -> bus_creator/99  "VINP_MCPressure_bar"
  bus_selector_1/85 -> UnitConverter_100/1  "<VINP_MCPressureV_flg>"
  UnitConverter_100/1 -> bus_creator/100  "VINP_MCPressureV_flg"
  bus_selector_1/86 -> UnitConverter_101/1  "<VINP_YawRate_degps>"
  UnitConverter_101/1 -> bus_creator/101  "VINP_YawRate_degps"
  bus_selector_1/87 -> UnitConverter_102/1  "<VINP_YawRateV_flg>"
  UnitConverter_102/1 -> bus_creator/102  "VINP_YawRateV_flg"
  bus_selector_1/88 -> UnitConverter_103/1  "<VINP_ActBrkLampSta_flg>"
  UnitConverter_103/1 -> bus_creator/103  "VINP_ActBrkLampSta_flg"
  bus_selector_1/89 -> UnitConverter_104/1  "<VINP_ESCADASSta_enum>"
  UnitConverter_104/1 -> bus_creator/104  "VINP_ESCADASSta_enum"
  bus_selector_1/90 -> UnitConverter_105/1  "<VINP_ESCAPSSta_enum>"
  UnitConverter_105/1 -> bus_creator/105  "VINP_ESCAPSSta_enum"
  bus_selector_1/91 -> UnitConverter_106/1  "<VINP_ESCStandstill_flg>"
  UnitConverter_106/1 -> bus_creator/106  "VINP_ESCStandstill_flg"
  bus_selector_1/92 -> UnitConverter_107/1  "<VINP_ESC7CSErr_flg>"
  UnitConverter_107/1 -> bus_creator/107  "VINP_ESC7CSErr_flg"
  bus_selector_1/93 -> UnitConverter_108/1  "<VINP_ESC7RCErr_flg>"
  UnitConverter_108/1 -> bus_creator/108  "VINP_ESC7RCErr_flg"
  bus_selector_1/94 -> UnitConverter_109/1  "<VINP_BrkPedalPos_pct>"
  UnitConverter_109/1 -> bus_creator/109  "VINP_BrkPedalPos_pct"
  bus_selector_1/95 -> UnitConverter_110/1  "<VINP_BrkPedalPosSta_flg>"
  UnitConverter_110/1 -> bus_creator/110  "VINP_BrkPedalPosSta_flg"
  bus_selector_1/96 -> UnitConverter_111/1  "<VINP_ESC7CS_enum>"
  UnitConverter_111/1 -> bus_creator/111  "VINP_ESC7CS_enum"
  bus_selector_1/97 -> UnitConverter_112/1  "<VINP_ESC7RC_enum>"
  UnitConverter_112/1 -> bus_creator/112  "VINP_ESC7RC_enum"
  bus_selector_1/98 -> UnitConverter_113/1  "<VINP_FrRBCActive_flg>"
  UnitConverter_113/1 -> bus_creator/113  "VINP_FrRBCActive_flg"
  bus_selector_1/99 -> UnitConverter_114/1  "<VINP_FrntAxlTrqReqBrk_Nm>"
  UnitConverter_114/1 -> bus_creator/114  "VINP_FrntAxlTrqReqBrk_Nm"
  bus_selector_1/100 -> UnitConverter_115/1  "<VINP_RDCActive_enum>"
  UnitConverter_115/1 -> bus_creator/115  "VINP_RDCActive_enum"
  bus_selector_1/101 -> UnitConverter_116/1  "<VINP_RearAxlTrqReqBrk_Nm>"
  UnitConverter_116/1 -> bus_creator/116  "VINP_RearAxlTrqReqBrk_Nm"
  bus_selector_1/102 -> UnitConverter_117/1  "<VINP_RrRBCActive_flg>"
  UnitConverter_117/1 -> bus_creator/117  "VINP_RrRBCActive_flg"
  bus_selector_1/103 -> UnitConverter_118/1  "<VINP_FCM2CSErr_flg>"
  UnitConverter_118/1 -> bus_creator/118  "VINP_FCM2CSErr_flg"
  bus_selector_1/104 -> UnitConverter_119/1  "<VINP_FCM2RCErr_flg>"
  UnitConverter_119/1 -> bus_creator/119  "VINP_FCM2RCErr_flg"
  bus_selector_1/105 -> UnitConverter_120/1  "<VINP_ACCRequiredAccel_mps2>"
  UnitConverter_120/1 -> bus_creator/120  "VINP_ACCRequiredAccel_mps2"
  bus_selector_1/106 -> UnitConverter_121/1  "<VINP_ACCVehHoldReq_flg>"
  UnitConverter_121/1 -> bus_creator/121  "VINP_ACCVehHoldReq_flg"
  bus_selector_1/107 -> UnitConverter_122/1  "<VINP_FCM2Checksum_enum>"
  UnitConverter_122/1 -> bus_creator/122  "VINP_FCM2Checksum_enum"
  bus_selector_1/108 -> UnitConverter_123/1  "<VINP_FCM2LifeCount_enum>"
  UnitConverter_123/1 -> bus_creator/123  "VINP_FCM2LifeCount_enum"
  bus_selector_1/109 -> UnitConverter_124/1  "<VINP_FCM3CSErr_flg>"
  UnitConverter_124/1 -> bus_creator/124  "VINP_FCM3CSErr_flg"
  bus_selector_1/110 -> UnitConverter_125/1  "<VINP_FCM3RCErr_flg>"
  UnitConverter_125/1 -> bus_creator/125  "VINP_FCM3RCErr_flg"
  bus_selector_1/111 -> UnitConverter_126/1  "<VINP_ACCObjDist_m>"
  UnitConverter_126/1 -> bus_creator/126  "VINP_ACCObjDist_m"
  bus_selector_1/112 -> UnitConverter_127/1  "<VINP_ACCObjRelSpd_mps>"
  UnitConverter_127/1 -> bus_creator/127  "VINP_ACCObjRelSpd_mps"
  bus_selector_1/113 -> UnitConverter_128/1  "<VINP_ADASForceIdle_flg>"
  UnitConverter_128/1 -> bus_creator/128  "VINP_ADASForceIdle_flg"
  bus_selector_1/114 -> UnitConverter_129/1  "<VINP_FCM3Checksum_enum>"
  UnitConverter_129/1 -> bus_creator/129  "VINP_FCM3Checksum_enum"
  bus_selector_1/115 -> UnitConverter_130/1  "<VINP_FCM3LifeCount_enum>"
  UnitConverter_130/1 -> bus_creator/130  "VINP_FCM3LifeCount_enum"
  bus_selector_1/116 -> UnitConverter_131/1  "<VINP_FCM4CSErr_flg>"
  UnitConverter_131/1 -> bus_creator/131  "VINP_FCM4CSErr_flg"
  bus_selector_1/117 -> UnitConverter_132/1  "<VINP_FCM4RCErr_flg>"
  UnitConverter_132/1 -> bus_creator/132  "VINP_FCM4RCErr_flg"
  bus_selector_1/118 -> UnitConverter_133/1  "<VINP_ACCSetSpeed_enum>"
  UnitConverter_133/1 -> bus_creator/133  "VINP_ACCSetSpeed_enum"
  bus_selector_1/119 -> UnitConverter_134/1  "<VINP_ACCSetSpeedDisp_enum>"
  UnitConverter_134/1 -> bus_creator/134  "VINP_ACCSetSpeedDisp_enum"
  bus_selector_1/120 -> UnitConverter_135/1  "<VINP_ADASACCSta_enum>"
  UnitConverter_135/1 -> bus_creator/135  "VINP_ADASACCSta_enum"
  bus_selector_1/121 -> UnitConverter_136/1  "<VINP_FCM4Checksum_enum>"
  UnitConverter_136/1 -> bus_creator/136  "VINP_FCM4Checksum_enum"
  bus_selector_1/122 -> UnitConverter_137/1  "<VINP_ForceLowBeam_enum>"
  UnitConverter_137/1 -> bus_creator/137  "VINP_ForceLowBeam_enum"
  bus_selector_1/123 -> UnitConverter_138/1  "<VINP_HazardWarningReq_flg>"
  UnitConverter_138/1 -> bus_creator/138  "VINP_HazardWarningReq_flg"
  bus_selector_1/124 -> UnitConverter_139/1  "<VINP_LeftTurnLightReq_flg>"
  UnitConverter_139/1 -> bus_creator/139  "VINP_LeftTurnLightReq_flg"
  bus_selector_1/125 -> UnitConverter_140/1  "<VINP_RightTurnLightReq_flg>"
  UnitConverter_140/1 -> bus_creator/140  "VINP_RightTurnLightReq_flg"
  bus_selector_1/126 -> UnitConverter_141/1  "<VINP_TargetType_enum>"
  UnitConverter_141/1 -> bus_creator/141  "VINP_TargetType_enum"
  bus_selector_1/127 -> UnitConverter_142/1  "<VINP_TimeGapLevel_enum>"
  UnitConverter_142/1 -> bus_creator/142  "VINP_TimeGapLevel_enum"
  bus_selector_1/128 -> UnitConverter_143/1  "<VINP_SRRBSDWarnL_enum>"
  UnitConverter_143/1 -> bus_creator/143  "VINP_SRRBSDWarnL_enum"
  bus_selector_1/129 -> UnitConverter_144/1  "<VINP_SRRBSDWarnR_enum>"
  UnitConverter_144/1 -> bus_creator/144  "VINP_SRRBSDWarnR_enum"
  bus_selector_1/130 -> UnitConverter_145/1  "<VINP_SRRODAWarnL_enum>"
  UnitConverter_145/1 -> bus_creator/145  "VINP_SRRODAWarnL_enum"
  bus_selector_1/131 -> UnitConverter_146/1  "<VINP_SRRODAWarnR_enum>"
  UnitConverter_146/1 -> bus_creator/146  "VINP_SRRODAWarnR_enum"
  [inp_CanValid_bus] -> bus_selector/1
  [inp_Hal_bus] -> bus_selector_1/1
  bus_creator/1 -> BINP_outputs/1
